simulink model "simulation_three_motors"  (R2022b)
settings: Solver=VariableStepAuto  StartTime=0.0  StopTime=10.0  RelTol=1e-3
settings Model: Creator=docto  LastModifiedBy=docto
settings ModelReferenceCC: EnableRefExpFcnMdlSchedulingChecks=on

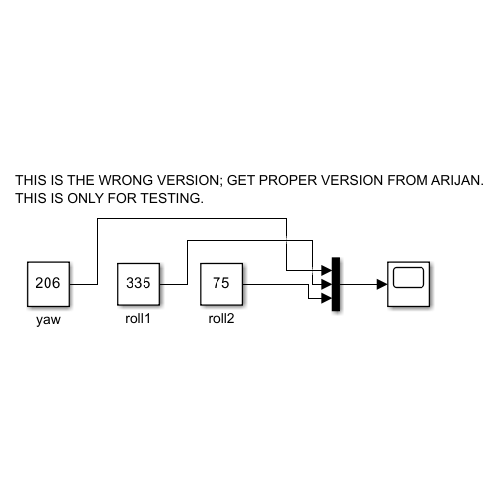
[thumbnail: Simulink's stored preview of the top-level diagram]
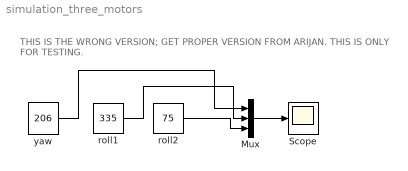
== system simulation_three_motors ==
  note: THIS IS THE WRONG VERSION; GET PROPER VERSION FROM ARIJAN.
      | THIS IS ONLY FOR TESTING.
  Mux : Mux  Inputs=3
  Scope : Scope
  roll1 : Constant  Value=335
  roll2 : Constant  Value=75
  yaw : Constant  Value=206
  wires:
  yaw/1 -> Mux/1
  roll1/1 -> Mux/2
  roll2/1 -> Mux/3
  Mux/1 -> Scope/1
